simulink model "lookup_nD_TestGen15"  (R2017b)
settings: Solver=FixedStepDiscrete  StartTime=0.0  StopTime=10.0  RelTol=1e-3
model workspace (MAT data in the model file):
  LUTObjLKnD15 = Simulink.LookupTable
  LUTObjLKnD15.Table = Simulink.lookuptable.Table
  LUTObjLKnD15.Table.Value = reshape([4 16 10 5 19 18 6 20 23 7 21 24 8 22 25 4 16 10 5 19 18 6 20 23 7 21 24 8 22 25], [2 5 3])
  LUTObjLKnD15.Table.Dimensions = [2 5 3]
  LUTObjLKnD15.Table.DataType = 'double'
  LUTObjLKnD15.Table.FieldName = 'Table'
  LUTObjLKnD15.Breakpoints(1) = Simulink.lookuptable.Breakpoint
  LUTObjLKnD15.Breakpoints(1).Value = [43.3441776625; 102.596007211]
  LUTObjLKnD15.Breakpoints(1).TunableSizeName = 'N1'
  LUTObjLKnD15.Breakpoints(1).Dimensions = [2 1]
  LUTObjLKnD15.Breakpoints(1).DataType = 'double'
  LUTObjLKnD15.Breakpoints(1).FieldName = 'BP1'
  LUTObjLKnD15.Breakpoints(2) = Simulink.lookuptable.Breakpoint
  LUTObjLKnD15.Breakpoints(2).Value = [13.5011354568; 27.5222953667; 56.8130592315; 65.0508060962; 102.036157926]
  LUTObjLKnD15.Breakpoints(2).TunableSizeName = 'N2'
  LUTObjLKnD15.Breakpoints(2).Dimensions = [5 1]
  LUTObjLKnD15.Breakpoints(2).DataType = 'double'
  LUTObjLKnD15.Breakpoints(2).FieldName = 'BP2'
  LUTObjLKnD15.Breakpoints(3) = Simulink.lookuptable.Breakpoint
  LUTObjLKnD15.Breakpoints(3).Value = [25.9211858801; 39.6875214095; 74.2617485445]
  LUTObjLKnD15.Breakpoints(3).TunableSizeName = 'N3'
  LUTObjLKnD15.Breakpoints(3).Dimensions = [3 1]
  LUTObjLKnD15.Breakpoints(3).DataType = 'double'
  LUTObjLKnD15.Breakpoints(3).FieldName = 'BP3'
  LUTObjLKnD15.SupportTunableSize = 0
  LUTObjLKnD15.StructTypeInfo = Simulink.lookuptable.StructTypeInfo
  LUTObjLKnD15.StructTypeInfo.Name = 'LUT'
  LUTObjLKnD15.StructTypeInfo.DataScope = 'Auto'
settings Model: Creator=ktrinh  LastModifiedBy=ktrinh
settings DebuggingCC: ParameterOverflowMsg=none

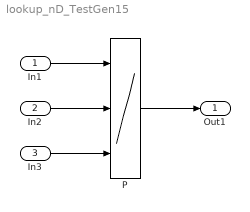
== system lookup_nD_TestGen15 ==
  In1 : Inport  OutMin=0  OutMax=127  PortDimensions=1
  In2 : Inport  Port=2  OutMin=0  OutMax=127
  In3 : Inport  Port=3  OutMin=0  OutMax=127
  P : Lookup_n-D  NumberOfTableDimensions=3  DataSpecification=Lookup table object  LookupTableObject=LUTObjLKnD15  BreakpointsForDimension3=[5, 7]  Table=reshape(repmat([4 5 6;16 19 20;10 18 23],1,2),[3,3,2])  InterpMethod=Nearest  ExtrapMethod=Clip  UseLastTableValue=on  InternalRulePriority=Speed  OutDataTypeStr=double  RndMeth=Convergent  SaturateOnIntegerOverflow=on  InputSameDT=on
  Out1 : Outport
  wires:
  In1/1 -> P/1
  In2/1 -> P/2
  In3/1 -> P/3
  P/1 -> Out1/1
